simulink model "Closed_loop_system"  (R2016b)
settings: Solver=VariableStepAuto  StartTime=0.0  StopTime=200  RelTol=1e-3
PreLoadFcn:
  | Driver=Simulink.Variant('passengerNumber==1')
  | Passengers=Simulink.Variant('passengerNumber==2')
  | Elephant=Simulink.Variant('passengerNumber==3')
  | 
  | passengerNumber=1
libraries: MeldasLibrary x4, simulink x1
settings Model: Creator=mulusoy  LastModifiedBy=mulusoy
settings DebuggingCC: SFUnconditionalPathOutOfParentDiag=warning  SFUnreachableStateOrJunctionDiag=warning  SFDanglingTransitionDiag=warning
settings CodeAppCC: CustomSymbolStrSimulinkFcn=$N
settings ConfigComp: CovMetricSettings=dswe

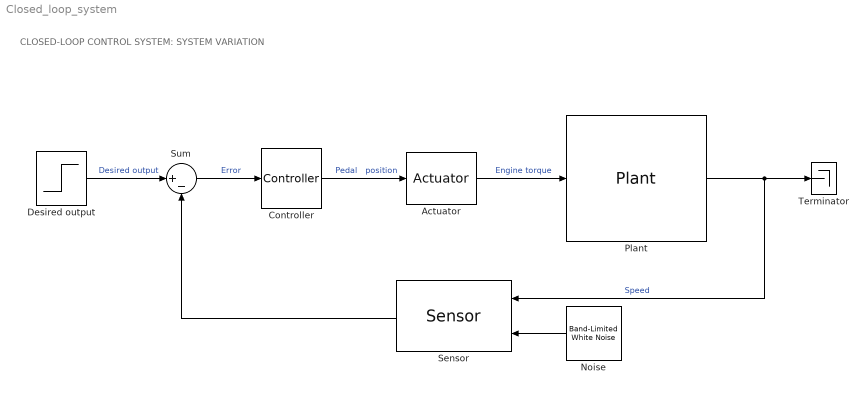
== system Closed_loop_system ==
  note: CLOSED-LOOP CONTROL SYSTEM: SYSTEM VARIATION
  Actuator : MeldasLibrary/Actuator  SystemSampleTime=-1
  Controller : MeldasLibrary/Controller  SystemSampleTime=-1
  Desired output : Step  Time=5  After=20  SampleTime=0
  Noise : simulink/Sources/Band-Limited White Noise  Cov=0.01  Ts=0.1  seed=[23341]
  Plant : MeldasLibrary/Plant  passengerNumber=Driver only
  Sensor : MeldasLibrary/Sensor  SystemSampleTime=-1
  Sum : Sum  Inputs=|+-
  Terminator : Terminator
  wires:
  Controller/1 -> Actuator/1  "Pedal   position"
  Actuator/1 -> Plant/1  "Engine torque"
  Plant/1 -> Sensor/1, Terminator/1  "Speed"
  Noise/1 -> Sensor/2
  Sensor/1 -> Sum/2
  Desired output/1 -> Sum/1  "Desired output"
  Sum/1 -> Controller/1  "Error"
